simulink model "pointing_spinstab"  (R2018b)
settings: Solver=VariableStepAuto  StartTime=0.0  StopTime=1000  RelTol=1e-3
settings Model: Creator=Stefano  LastModifiedBy=aloisia
settings SolverCC: DecoupledContinuousIntegration=on  MinimalZcImpactIntegration=on
settings DebuggingCC: LibraryContextMissingDiagnostic=none
settings SFSimCC: SimUseLocalCustomCode=off
settings RTWCC: RTWUseLocalCustomCode=off

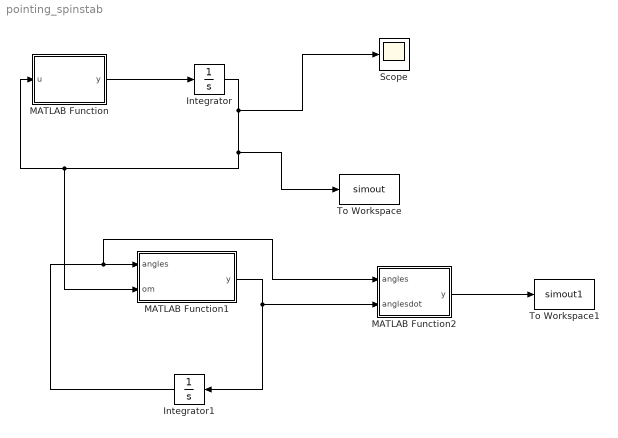
== system pointing_spinstab ==
  Integrator : Integrator  InitialCondition=[0.1; 0.05; 15*pi/180]
  Integrator1 : Integrator  InitialCondition=[0.1;0.2;0.3]
  MATLAB Function : MATLAB Function  TreatAsAtomicUnit=on
  MATLAB Function1 : MATLAB Function  TreatAsAtomicUnit=on
  MATLAB Function2 : MATLAB Function  TreatAsAtomicUnit=on
  Scope : Scope
  To Workspace : ToWorkspace  VariableName=simout  SampleTime=-1
  To Workspace1 : ToWorkspace  VariableName=simout1  SampleTime=-1
  wires:
  MATLAB Function/1(y) -> Integrator/1
  Integrator/1 -> Scope/1, To Workspace/1, MATLAB Function1/2(om), MATLAB Function/1(u)
  MATLAB Function1/1(y) -> Integrator1/1, MATLAB Function2/2(anglesdot)
  Integrator1/1 -> MATLAB Function2/1(angles), MATLAB Function1/1(angles)
  MATLAB Function2/1(y) -> To Workspace1/1

== matlab function pointing_spinstab/MATLAB Function1 ==
  data: angles input; y output; om input

function y = fcn(angles,om)

% This function provides the calculation of A by using 
% Phi, theta, psi and omega.Radiants
phi = angles(1);
theta = angles(2);
psi = angles(3);

phidot = (om(1)*cos(psi) - om(2)*sin(psi)) / cos(theta);
thetadot = om(2)*cos(psi) + om(1)*sin(psi);
psidot = om(3) - (om(1)*cos(psi) - om(2)*sin(psi))* sin(theta)/cos(theta);
anglesdot = [phidot; thetadot; psidot];

y = anglesdot;
end

== matlab function pointing_spinstab/MATLAB Function ==
  data: u input; y output
function y = fcn(u)
%First laboratory

%Datas
Ix=0.01;
Iy=0.05;
Iz=0.07;

omx=u(1);
omy=u(2);
omz=u(3);

%Formula
omxdot=(Iy-Iz)/Ix*omy*omz;
omydot=(Iz-Ix)/Iy*omx*omz;
omzdot=(Ix-Iy)/Iz*omy*omx;

y=[omxdot; omydot; omzdot];

u=y;

end

== matlab function pointing_spinstab/MATLAB Function2 ==
  data: angles input; y output; anglesdot input
function y = fcn(angles,anglesdot)

phi = angles(1);
theta = angles(2);
psi = angles(3);

A = [cos(psi)*cos(theta) cos(psi)*sin(theta)*sin(phi)+cos(phi)*sin(psi) -cos(psi)*sin(theta)*cos(phi)+sin(psi)*sin(phi);...
    -sin(psi)*cos(theta) -sin(psi)*sin(theta)*sin(phi)+cos(psi)*cos(phi) sin(psi)*sin(theta)*cos(phi)+cos(psi)*sin(phi);...
    sin(theta) -cos(theta)*sin(phi) cos(theta)*cos(phi)];
om = A*anglesdot;

y=A'*[0 0 1]';
end
